simulink model "torqueBalancingR2015a"  (Simulink 8.5)
settings: Solver=FixedStepDiscrete  StartTime=0.0  StopTime="CONFIG.SIMULATION_TIME "  FixedStep=CONFIG.Ts  RelTol=1e-3
InitFcn:
  | cd(fileparts(which(bdroot)));
  | initTorqueBalancing;
values from neighbouring files (symbols this model uses):
  WBT_robotName = 'iCub'    [initTorqueBalancing.m]
undefined symbols (not defined in the file or in its folder): bVectorConstraints, CONFIG, ConstraintsMatrix, DiscIntNeverNeededParam, gain, references, reg, ROBOT_DOF, ROBOT_DOF_FOR_SIMULINK, sat, SM, sm
libraries: WBToolboxLibrary x126, simulink x6
(part 2 of 3)

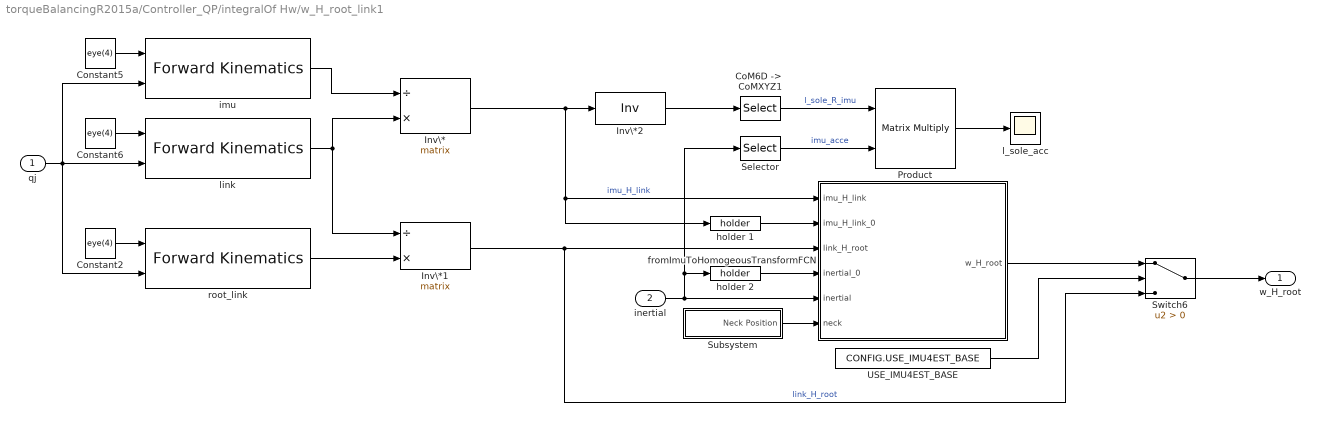
== system torqueBalancingR2015a/Controller_QP/integralOf Hw/w_H_root_link1 ==
  qj : Inport
  inertial : Inport  Port=2
  "CoM6D ->  CoMXYZ1" : Selector  NumberOfDimensions=2  InputPortWidth=7  IndexOptions=Index vector (dialog),Index vector (dialog)  Indices=[1 2 3],[1 2 3]  OutputSizes=1,1
  Constant2 : Constant  Value=eye(4)
  Constant5 : Constant  Value=eye(4)
  Constant6 : Constant  Value=eye(4)
  Inv\* : Product  Inputs=/*  Multiplication=Matrix(*)
  Inv\*1 : Product  Inputs=/*  Multiplication=Matrix(*)
  Inv\*2 : Product  Inputs=/  Multiplication=Matrix(*)
  Product : Product  Multiplication=Matrix(*)
  Selector : Selector  InputPortWidth=12  IndexOptions=Index vector (dialog)  Indices=[4 5 6 ]  OutputSizes=1
  Subsystem : Subsystem
  Switch6 : Switch  Criteria=u2 > Threshold
  USE_IMU4EST_BASE : Constant  Value=CONFIG.USE_IMU4EST_BASE
  fromImuToHomogeousTransformFCN : MATLAB Function  TreatAsAtomicUnit=on
      settings: PermitHierarchicalResolution=ParametersOnly
  holder 1 : WBToolboxLibrary/Utilities/holder 
  holder 2 : WBToolboxLibrary/Utilities/holder 
  imu : WBToolboxLibrary/wholeBodyModel/Kinematics/Forward Kinematics  frameName='imu_frame'  robotName=WBT_robotName  localName=WBT_modelName  wbiFile=WBT_wbiFilename  wbiList=WBT_wbiList
  l_sole_acc : Scope
      settings: TimeRange=auto  LimitDataPoints=on  MaxDataPoints=5000  SaveToWorkspace=off  SaveName=ScopeData  YMin=-10  YMax=10  SampleTime=-1  DataFormat=Array
  link : WBToolboxLibrary/wholeBodyModel/Kinematics/Forward Kinematics  frameName=link_name  robotName=WBT_robotName  localName=WBT_modelName  wbiFile=WBT_wbiFilename  wbiList=WBT_wbiList
  root_link : WBToolboxLibrary/wholeBodyModel/Kinematics/Forward Kinematics  frameName='root_link'  robotName=WBT_robotName  localName=WBT_modelName  wbiFile=WBT_wbiFilename  wbiList=WBT_wbiList
  w_H_root : Outport
  wires:
  Constant5/1 -> imu/1
  Inv\*/1 -> holder 1/1, fromImuToHomogeousTransformFCN/1(imu_H_link), Inv\*2/1  "imu_H_link"
  imu/1 -> Inv\*/1
  Constant6/1 -> link/1
  Inv\*1/1 -> Switch6/3, fromImuToHomogeousTransformFCN/3(link_H_root)  "link_H_root"
  link/1 -> Inv\*1/1, Inv\*/2
  inertial/1 -> Selector/1, holder 2/1, fromImuToHomogeousTransformFCN/5(inertial)
  Switch6/1 -> w_H_root/1
  USE_IMU4EST_BASE/1 -> Switch6/2
  fromImuToHomogeousTransformFCN/1(w_H_root) -> Switch6/1
  Constant2/1 -> root_link/1
  qj/1 -> root_link/2, link/2, imu/2
  root_link/1 -> Inv\*1/2
  holder 1/1 -> fromImuToHomogeousTransformFCN/2(imu_H_link_0)
  holder 2/1 -> fromImuToHomogeousTransformFCN/4(inertial_0)
  Inv\*2/1 -> "CoM6D ->  CoMXYZ1"/1
  "CoM6D ->  CoMXYZ1"/1 -> Product/1  "l_sole_R_imu"
  Selector/1 -> Product/2  "imu_acce"
  Product/1 -> l_sole_acc/1
  Subsystem/1(Neck Position) -> fromImuToHomogeousTransformFCN/6(neck)

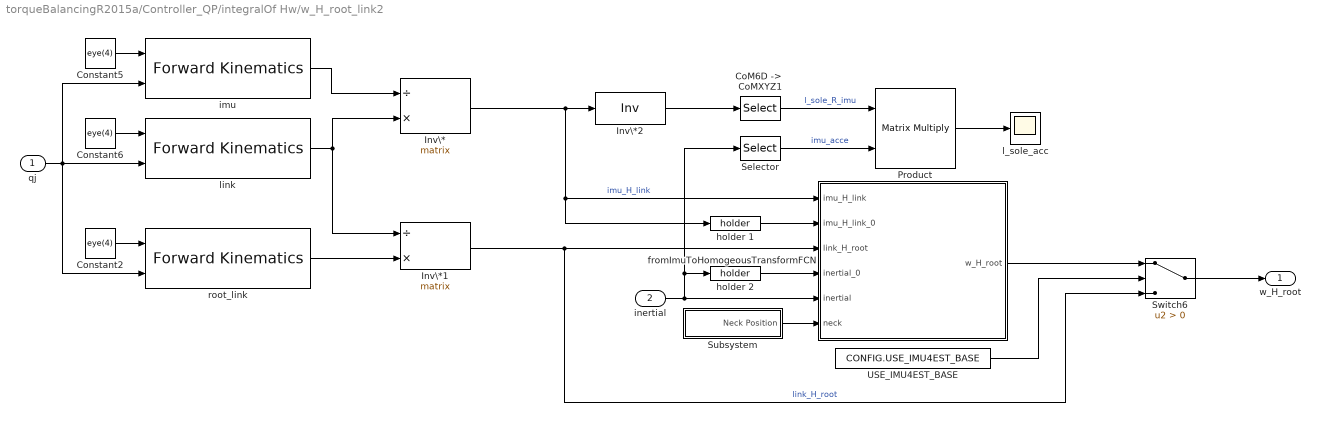
== system torqueBalancingR2015a/Controller_QP/integralOf Hw/w_H_root_link2 ==
  qj : Inport
  inertial : Inport  Port=2
  "CoM6D ->  CoMXYZ1" : Selector  NumberOfDimensions=2  InputPortWidth=7  IndexOptions=Index vector (dialog),Index vector (dialog)  Indices=[1 2 3],[1 2 3]  OutputSizes=1,1
  Constant2 : Constant  Value=eye(4)
  Constant5 : Constant  Value=eye(4)
  Constant6 : Constant  Value=eye(4)
  Inv\* : Product  Inputs=/*  Multiplication=Matrix(*)
  Inv\*1 : Product  Inputs=/*  Multiplication=Matrix(*)
  Inv\*2 : Product  Inputs=/  Multiplication=Matrix(*)
  Product : Product  Multiplication=Matrix(*)
  Selector : Selector  InputPortWidth=12  IndexOptions=Index vector (dialog)  Indices=[4 5 6 ]  OutputSizes=1
  Subsystem : Subsystem
  Switch6 : Switch  Criteria=u2 > Threshold
  USE_IMU4EST_BASE : Constant  Value=CONFIG.USE_IMU4EST_BASE
  fromImuToHomogeousTransformFCN : MATLAB Function  TreatAsAtomicUnit=on
      settings: PermitHierarchicalResolution=ParametersOnly
  holder 1 : WBToolboxLibrary/Utilities/holder 
  holder 2 : WBToolboxLibrary/Utilities/holder 
  imu : WBToolboxLibrary/wholeBodyModel/Kinematics/Forward Kinematics  frameName='imu_frame'  robotName=WBT_robotName  localName=WBT_modelName  wbiFile=WBT_wbiFilename  wbiList=WBT_wbiList
  l_sole_acc : Scope
      settings: TimeRange=auto  LimitDataPoints=on  MaxDataPoints=5000  SaveToWorkspace=off  SaveName=ScopeData  YMin=-10  YMax=10  SampleTime=-1  DataFormat=Array
  link : WBToolboxLibrary/wholeBodyModel/Kinematics/Forward Kinematics  frameName=link_name  robotName=WBT_robotName  localName=WBT_modelName  wbiFile=WBT_wbiFilename  wbiList=WBT_wbiList
  root_link : WBToolboxLibrary/wholeBodyModel/Kinematics/Forward Kinematics  frameName='root_link'  robotName=WBT_robotName  localName=WBT_modelName  wbiFile=WBT_wbiFilename  wbiList=WBT_wbiList
  w_H_root : Outport
  wires:
  Constant5/1 -> imu/1
  Inv\*/1 -> holder 1/1, fromImuToHomogeousTransformFCN/1(imu_H_link), Inv\*2/1  "imu_H_link"
  imu/1 -> Inv\*/1
  Constant6/1 -> link/1
  Inv\*1/1 -> Switch6/3, fromImuToHomogeousTransformFCN/3(link_H_root)  "link_H_root"
  link/1 -> Inv\*1/1, Inv\*/2
  inertial/1 -> Selector/1, holder 2/1, fromImuToHomogeousTransformFCN/5(inertial)
  Switch6/1 -> w_H_root/1
  USE_IMU4EST_BASE/1 -> Switch6/2
  fromImuToHomogeousTransformFCN/1(w_H_root) -> Switch6/1
  Constant2/1 -> root_link/1
  qj/1 -> root_link/2, link/2, imu/2
  root_link/1 -> Inv\*1/2
  holder 1/1 -> fromImuToHomogeousTransformFCN/2(imu_H_link_0)
  holder 2/1 -> fromImuToHomogeousTransformFCN/4(inertial_0)
  Inv\*2/1 -> "CoM6D ->  CoMXYZ1"/1
  "CoM6D ->  CoMXYZ1"/1 -> Product/1  "l_sole_R_imu"
  Selector/1 -> Product/2  "imu_acce"
  Product/1 -> l_sole_acc/1
  Subsystem/1(Neck Position) -> fromImuToHomogeousTransformFCN/6(neck)

== system torqueBalancingR2015a/State Machine/Internal coordinator/nu ==
  qj : Inport
  w_H_b : Inport  Port=2
  "constraints " : Inport  Port=3
  Get Estimate : WBToolboxLibrary/wholeBodyStates/Get Estimate  estimateType=Joints Velocity  robotName=WBT_robotName  localName=WBT_modelName  wbiFile=WBT_wbiFilename  wbiList=WBT_wbiList
  Jacobian l_sole : WBToolboxLibrary/wholeBodyModel/Jacobians/Jacobian  frameName='l_sole'  robotName=WBT_robotName  localName=WBT_modelName  wbiFile=WBT_wbiFilename  wbiList=WBT_wbiList
  Jacobian r_sole : WBToolboxLibrary/wholeBodyModel/Jacobians/Jacobian  frameName='r_sole'  robotName=WBT_robotName  localName=WBT_modelName  wbiFile=WBT_wbiFilename  wbiList=WBT_wbiList
  MATLAB Function : MATLAB Function  TreatAsAtomicUnit=on
      settings: PermitHierarchicalResolution=ParametersOnly
  Mux : Mux  Inputs=2
  vb + Dqj : Outport
  wires:
  Get Estimate/1 -> MATLAB Function/4(qD), Mux/2
  Mux/1 -> vb + Dqj/1
  Jacobian r_sole/1 -> MATLAB Function/2(JcRightFoot)
  "constraints "/1 -> MATLAB Function/3(activeFeetConstraints)
  MATLAB Function/1(y) -> Mux/1
  Jacobian l_sole/1 -> MATLAB Function/1(JcLeftFoot)
  qj/1 -> Jacobian l_sole/2, Jacobian r_sole/2
  w_H_b/1 -> Jacobian r_sole/1, Jacobian l_sole/1

== system torqueBalancingR2015a/State Machine/Internal coordinator/refGen ==
  xCom(0) : Inport
  qj(0) : Inport  Port=2
  Enable : EnablePort
  Clock1 : Clock
  refGenFCN : MATLAB Function  TreatAsAtomicUnit=on
      settings: PermitHierarchicalResolution=ParametersOnly
  qDes : Outport
  CoMrefs : Outport  Port=2
  wires:
  refGenFCN/2(desired_x_dx_ddx_CoM) -> CoMrefs/1
  xCom(0)/1 -> refGenFCN/1(xCom0)
  Clock1/1 -> refGenFCN/3(t)
  qj(0)/1 -> refGenFCN/2(q0)
  refGenFCN/1(qDes) -> qDes/1

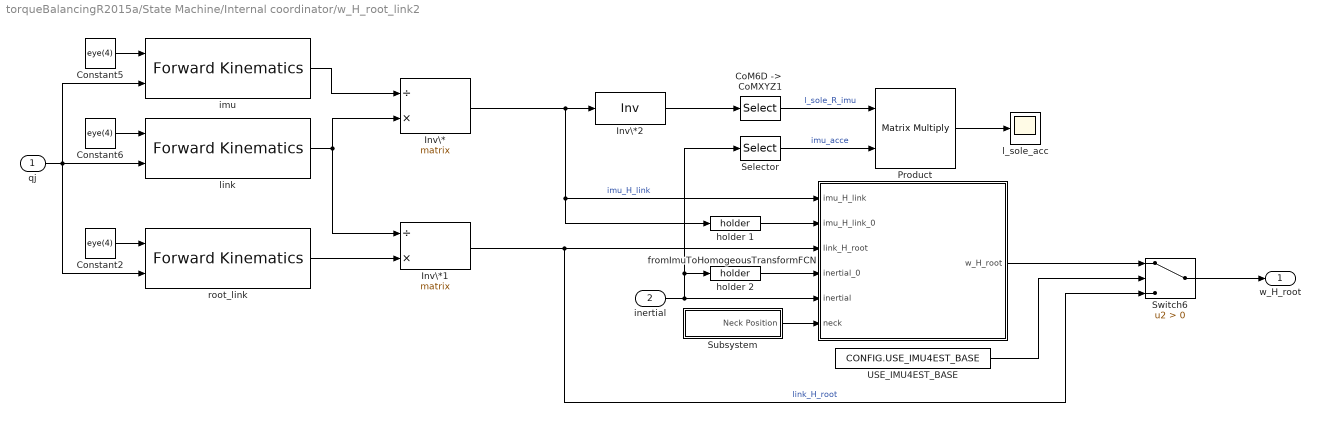
== system torqueBalancingR2015a/State Machine/Internal coordinator/w_H_root_link2 ==
  qj : Inport
  inertial : Inport  Port=2
  "CoM6D ->  CoMXYZ1" : Selector  NumberOfDimensions=2  InputPortWidth=7  IndexOptions=Index vector (dialog),Index vector (dialog)  Indices=[1 2 3],[1 2 3]  OutputSizes=1,1
  Constant2 : Constant  Value=eye(4)
  Constant5 : Constant  Value=eye(4)
  Constant6 : Constant  Value=eye(4)
  Inv\* : Product  Inputs=/*  Multiplication=Matrix(*)
  Inv\*1 : Product  Inputs=/*  Multiplication=Matrix(*)
  Inv\*2 : Product  Inputs=/  Multiplication=Matrix(*)
  Product : Product  Multiplication=Matrix(*)
  Selector : Selector  InputPortWidth=12  IndexOptions=Index vector (dialog)  Indices=[4 5 6 ]  OutputSizes=1
  Subsystem : Subsystem
  Switch6 : Switch  Criteria=u2 > Threshold
  USE_IMU4EST_BASE : Constant  Value=CONFIG.USE_IMU4EST_BASE
  fromImuToHomogeousTransformFCN : MATLAB Function  TreatAsAtomicUnit=on
      settings: PermitHierarchicalResolution=ParametersOnly
  holder 1 : WBToolboxLibrary/Utilities/holder 
  holder 2 : WBToolboxLibrary/Utilities/holder 
  imu : WBToolboxLibrary/wholeBodyModel/Kinematics/Forward Kinematics  frameName='imu_frame'  robotName=WBT_robotName  localName=WBT_modelName  wbiFile=WBT_wbiFilename  wbiList=WBT_wbiList
  l_sole_acc : Scope
      settings: TimeRange=auto  LimitDataPoints=on  MaxDataPoints=5000  SaveToWorkspace=off  SaveName=ScopeData  YMin=-10  YMax=10  SampleTime=-1  DataFormat=Array
  link : WBToolboxLibrary/wholeBodyModel/Kinematics/Forward Kinematics  frameName=link_name  robotName=WBT_robotName  localName=WBT_modelName  wbiFile=WBT_wbiFilename  wbiList=WBT_wbiList
  root_link : WBToolboxLibrary/wholeBodyModel/Kinematics/Forward Kinematics  frameName='root_link'  robotName=WBT_robotName  localName=WBT_modelName  wbiFile=WBT_wbiFilename  wbiList=WBT_wbiList
  w_H_root : Outport
  wires:
  Constant5/1 -> imu/1
  Inv\*/1 -> holder 1/1, fromImuToHomogeousTransformFCN/1(imu_H_link), Inv\*2/1  "imu_H_link"
  imu/1 -> Inv\*/1
  Constant6/1 -> link/1
  Inv\*1/1 -> Switch6/3, fromImuToHomogeousTransformFCN/3(link_H_root)  "link_H_root"
  link/1 -> Inv\*1/1, Inv\*/2
  inertial/1 -> Selector/1, holder 2/1, fromImuToHomogeousTransformFCN/5(inertial)
  Switch6/1 -> w_H_root/1
  USE_IMU4EST_BASE/1 -> Switch6/2
  fromImuToHomogeousTransformFCN/1(w_H_root) -> Switch6/1
  Constant2/1 -> root_link/1
  qj/1 -> root_link/2, link/2, imu/2
  root_link/1 -> Inv\*1/2
  holder 1/1 -> fromImuToHomogeousTransformFCN/2(imu_H_link_0)
  holder 2/1 -> fromImuToHomogeousTransformFCN/4(inertial_0)
  Inv\*2/1 -> "CoM6D ->  CoMXYZ1"/1
  "CoM6D ->  CoMXYZ1"/1 -> Product/1  "l_sole_R_imu"
  Selector/1 -> Product/2  "imu_acce"
  Product/1 -> l_sole_acc/1
  Subsystem/1(Neck Position) -> fromImuToHomogeousTransformFCN/6(neck)

== system torqueBalancingR2015a/State Machine/Internal coordinator/xCom ==
  w_H_b : Inport
  qj : Inport  Port=2
  "CoM6D ->  CoMXYZ2" : Selector  NumberOfDimensions=2  InputPortWidth=7  IndexOptions=Index vector (dialog),Index vector (dialog)  Indices=[1 2 3],[4]  OutputSizes=1,1
  com : WBToolboxLibrary/wholeBodyModel/Kinematics/Forward Kinematics  frameName='com'  robotName=WBT_robotName  localName=WBT_modelName  wbiFile=WBT_wbiFilename  wbiList=WBT_wbiList
  xCom : Outport
  wires:
  qj/1 -> com/2
  "CoM6D ->  CoMXYZ2"/1 -> xCom/1
  com/1 -> "CoM6D ->  CoMXYZ2"/1
  w_H_b/1 -> com/1

== system torqueBalancingR2015a/State Machine/State Machine Walking/Visualise external wrenches   ==
  wL_WBDT : Inport
  wR_WBDT : Inport  Port=2
  Enable : EnablePort
  Constant : Constant  Value=sm.wrench.thresholdContactOn
  Constant2 : Constant  Value=sm.wrench.thresholdContactOff
  left foot ext wrench : Scope  NumInputPorts=3
      settings: TimeRange=auto  LimitDataPoints=on  MaxDataPoints=5000  SaveToWorkspace=off  SaveName=ScopeData  YMin=-47.59687~15.00000~75.00000  YMax=331.67201~35.00000~95.00000  SampleTime=-1  DataFormat=Array
  right foot ext wrench : Scope  NumInputPorts=3
      settings: TimeRange=auto  LimitDataPoints=on  MaxDataPoints=5000  SaveToWorkspace=off  SaveName=ScopeData  YMin=-42.03924~15.00000~75.00000  YMax=233.22188~35.00000~95.00000  SampleTime=-1  DataFormat=Array
  wires:
  Constant/1 -> right foot ext wrench/2, left foot ext wrench/2  "thresholdContactOn"
  wR_WBDT/1 -> right foot ext wrench/1  "wR_WBDT"
  wL_WBDT/1 -> left foot ext wrench/1  "wL_WBDT"
  Constant2/1 -> right foot ext wrench/3, left foot ext wrench/3  "thresholdContactOff"

== system torqueBalancingR2015a/State Machine/State Machine Walking/nu ==
  w_H_b : Inport
  "constraints " : Inport  Port=2
  qj : Inport  Port=3
  Get Estimate : WBToolboxLibrary/wholeBodyStates/Get Estimate  estimateType=Joints Velocity  robotName=WBT_robotName  localName=WBT_modelName  wbiFile=WBT_wbiFilename  wbiList=WBT_wbiList
  Jacobian l_sole : WBToolboxLibrary/wholeBodyModel/Jacobians/Jacobian  frameName='l_sole'  robotName=WBT_robotName  localName=WBT_modelName  wbiFile=WBT_wbiFilename  wbiList=WBT_wbiList
  Jacobian r_sole : WBToolboxLibrary/wholeBodyModel/Jacobians/Jacobian  frameName='r_sole'  robotName=WBT_robotName  localName=WBT_modelName  wbiFile=WBT_wbiFilename  wbiList=WBT_wbiList
  MATLAB Function : MATLAB Function  TreatAsAtomicUnit=on
      settings: PermitHierarchicalResolution=ParametersOnly
  Mux : Mux  Inputs=2
  vb + Dqj : Outport
  wires:
  Get Estimate/1 -> MATLAB Function/4(qD), Mux/2
  Mux/1 -> vb + Dqj/1
  Jacobian r_sole/1 -> MATLAB Function/2(JcRightFoot)
  "constraints "/1 -> MATLAB Function/3(activeFeetConstraints)
  MATLAB Function/1(y) -> Mux/1
  Jacobian l_sole/1 -> MATLAB Function/1(JcLeftFoot)
  qj/1 -> Jacobian l_sole/2, Jacobian r_sole/2
  w_H_b/1 -> Jacobian r_sole/1, Jacobian l_sole/1

== system torqueBalancingR2015a/State Machine/State Machine Walking/visualise inertial ==
  jointAngles : Inport
  inertial : Inport  Port=2
  Enable : EnablePort
  Inv\* : Product  Inputs=/*  Multiplication=Matrix(*)
  Inv\*1 : Product  Inputs=/*  Multiplication=Matrix(*)
  Visualize hom transf1 : Subsystem
  Visualize hom transf2 : Subsystem
  Visualize hom transf3 : Subsystem
  Visualize hom transf4 : Subsystem
  Visualize hom transf5 : Subsystem
  Visualize hom transf7 : Subsystem
  "inertial -> rpy" : Selector  InputPortWidth=12  IndexOptions=Index vector (dialog)  Indices=[1 2 3]  OutputSizes=1
  l_sole_H_root_link1 : Subsystem  mask{link_name='l_sole'}
  l_sole_H_root_link2 : Subsystem  mask{link_name='l_sole'}
  rpy : Scope
      settings: TimeRange=auto  LimitDataPoints=on  MaxDataPoints=5000  SaveToWorkspace=off  SaveName=ScopeData  YMin=-10  YMax=10  SampleTime=-1  DataFormat=Array
  w_H_root_link1 : Subsystem  mask{link_name='r_sole'}
      mask prompts: link_name "link name"
      mask help:
      | This block evaluates the homogeneous transformation between the world and the root link, i.e. ^wH_b. It assumes that the link specified by the variable 'link_name' has a constant position
      | w.r.t. an inertial frame, but it can rotate arbitrarily. This rotation is retrived from the IMU sensor.
      mask Display:
      | str = strrep(link_name, '_','\_');
      | port_label('output',1,['{}^{',str '}H_{root}'],'texmode','on')
      | clear str;
      | 
      | port_label('input',1,'q_j','texmode','on')
      | 
      | port_label('input',2,'inertial','texmode','on')
  w_H_root_link2 : Subsystem  mask{link_name='l_sole'}
      mask prompts: link_name "link name"
      mask help:
      | This block evaluates the homogeneous transformation between the world and the root link, i.e. ^wH_b. It assumes that the link specified by the variable 'link_name' has a constant position
      | w.r.t. an inertial frame, but it can rotate arbitrarily. This rotation is retrived from the IMU sensor.
      mask Display:
      | str = strrep(link_name, '_','\_');
      | port_label('output',1,['{}^{',str '}H_{root}'],'texmode','on')
      | clear str;
      | 
      | port_label('input',1,'q_j','texmode','on')
      | 
      | port_label('input',2,'inertial','texmode','on')
  wires:
  inertial/1 -> w_H_root_link1/2(inertial), w_H_root_link2/2(inertial), "inertial -> rpy"/1
  jointAngles/1 -> l_sole_H_root_link2/1(qj), l_sole_H_root_link1/1(qj), w_H_root_link1/1(qj), w_H_root_link2/1(qj)
  l_sole_H_root_link2/1(link_name_H_root_link) -> Visualize hom transf7/1(H), Inv\*/1  "l_sole_H_root_link"
  Inv\*/1 -> Visualize hom transf4/1(H)
  w_H_root_link2/1(w_H_root) -> Inv\*/2, Visualize hom transf1/1(H)
  "inertial -> rpy"/1 -> rpy/1
  l_sole_H_root_link1/1(link_name_H_root_link) -> Visualize hom transf2/1(H), Inv\*1/1  "r_sole_H_root_link"
  Inv\*1/1 -> Visualize hom transf3/1(H)
  w_H_root_link1/1(w_H_root) -> Inv\*1/2, Visualize hom transf5/1(H)

== system torqueBalancingR2015a/State Machine/State Machine Walking/xCom2 ==
  qj : Inport
  w_H_b : Inport  Port=2
  "CoM6D ->  CoMXYZ2" : Selector  NumberOfDimensions=2  InputPortWidth=7  IndexOptions=Index vector (dialog),Index vector (dialog)  Indices=[1 2 3],[4]  OutputSizes=1,1
  com : WBToolboxLibrary/wholeBodyModel/Kinematics/Forward Kinematics  frameName='com'  robotName=WBT_robotName  localName=WBT_modelName  wbiFile=WBT_wbiFilename  wbiList=WBT_wbiList
  xCoM : Outport
  wires:
  qj/1 -> com/2
  "CoM6D ->  CoMXYZ2"/1 -> xCoM/1
  com/1 -> "CoM6D ->  CoMXYZ2"/1
  w_H_b/1 -> com/1

== system torqueBalancingR2015a/State Machine/State Machine Yoga/Visualise external wrenches   ==
  wL_WBDT : Inport
  wR_WBDT : Inport  Port=2
  Enable : EnablePort
  Constant : Constant  Value=sm.wrench.thresholdContactOn
  Constant2 : Constant  Value=sm.wrench.thresholdContactOff
  left foot ext wrench : Scope  NumInputPorts=3
      settings: TimeRange=auto  LimitDataPoints=on  MaxDataPoints=5000  SaveToWorkspace=off  SaveName=ScopeData  YMin=-10~-10~-10  YMax=10~10~10  SampleTime=-1  DataFormat=Array
  right foot ext wrench : Scope  NumInputPorts=3
      settings: TimeRange=auto  LimitDataPoints=on  MaxDataPoints=5000  SaveToWorkspace=off  SaveName=ScopeData  YMin=-10~-10~-10  YMax=10~10~10  SampleTime=-1  DataFormat=Array
  wires:
  Constant/1 -> left foot ext wrench/2, right foot ext wrench/2  "thresholdContactOn"
  wR_WBDT/1 -> right foot ext wrench/1  "wR_WBDT"
  wL_WBDT/1 -> left foot ext wrench/1  "wL_WBDT"
  Constant2/1 -> left foot ext wrench/3, right foot ext wrench/3  "thresholdContactOff"

== system torqueBalancingR2015a/State Machine/State Machine Yoga/nu ==
  qj : Inport
  w_H_b : Inport  Port=2
  "constraints " : Inport  Port=3
  Get Estimate : WBToolboxLibrary/wholeBodyStates/Get Estimate  estimateType=Joints Velocity  robotName=WBT_robotName  localName=WBT_modelName  wbiFile=WBT_wbiFilename  wbiList=WBT_wbiList
  Jacobian l_sole : WBToolboxLibrary/wholeBodyModel/Jacobians/Jacobian  frameName='l_sole'  robotName=WBT_robotName  localName=WBT_modelName  wbiFile=WBT_wbiFilename  wbiList=WBT_wbiList
  Jacobian r_sole : WBToolboxLibrary/wholeBodyModel/Jacobians/Jacobian  frameName='r_sole'  robotName=WBT_robotName  localName=WBT_modelName  wbiFile=WBT_wbiFilename  wbiList=WBT_wbiList
  MATLAB Function : MATLAB Function  TreatAsAtomicUnit=on
      settings: PermitHierarchicalResolution=ParametersOnly
  Mux : Mux  Inputs=2
  vb + Dqj : Outport
  wires:
  Get Estimate/1 -> MATLAB Function/4(qD), Mux/2
  Mux/1 -> vb + Dqj/1
  Jacobian r_sole/1 -> MATLAB Function/2(JcRightFoot)
  "constraints "/1 -> MATLAB Function/3(activeFeetConstraints)
  MATLAB Function/1(y) -> Mux/1
  Jacobian l_sole/1 -> MATLAB Function/1(JcLeftFoot)
  qj/1 -> Jacobian l_sole/2, Jacobian r_sole/2
  w_H_b/1 -> Jacobian r_sole/1, Jacobian l_sole/1

== system torqueBalancingR2015a/State Machine/State Machine Yoga/visualise inertial ==
  jointAngles : Inport
  inertial : Inport  Port=2
  Enable : EnablePort
  Inv\* : Product  Inputs=/*  Multiplication=Matrix(*)
  Inv\*1 : Product  Inputs=/*  Multiplication=Matrix(*)
  Visualize hom transf1 : Subsystem
  Visualize hom transf2 : Subsystem
  Visualize hom transf3 : Subsystem
  Visualize hom transf4 : Subsystem
  Visualize hom transf5 : Subsystem
  Visualize hom transf7 : Subsystem
  "inertial -> rpy" : Selector  InputPortWidth=12  IndexOptions=Index vector (dialog)  Indices=[1 2 3]  OutputSizes=1
  l_sole_H_root_link1 : Subsystem  mask{link_name='l_sole'}
  l_sole_H_root_link2 : Subsystem  mask{link_name='l_sole'}
  rpy : Scope
      settings: TimeRange=auto  LimitDataPoints=on  MaxDataPoints=5000  SaveToWorkspace=off  SaveName=ScopeData  YMin=-10  YMax=10  SampleTime=-1  DataFormat=Array
  w_H_root_link1 : Subsystem  mask{link_name='r_sole'}
      mask prompts: link_name "link name"
      mask help:
      | This block evaluates the homogeneous transformation between the world and the root link, i.e. ^wH_b. It assumes that the link specified by the variable 'link_name' has a constant position
      | w.r.t. an inertial frame, but it can rotate arbitrarily. This rotation is retrived from the IMU sensor.
      mask Display:
      | str = strrep(link_name, '_','\_');
      | port_label('output',1,['{}^{',str '}H_{root}'],'texmode','on')
      | clear str;
      | 
      | port_label('input',1,'q_j','texmode','on')
      | 
      | port_label('input',2,'inertial','texmode','on')
  w_H_root_link2 : Subsystem  mask{link_name='l_sole'}
      mask prompts: link_name "link name"
      mask help:
      | This block evaluates the homogeneous transformation between the world and the root link, i.e. ^wH_b. It assumes that the link specified by the variable 'link_name' has a constant position
      | w.r.t. an inertial frame, but it can rotate arbitrarily. This rotation is retrived from the IMU sensor.
      mask Display:
      | str = strrep(link_name, '_','\_');
      | port_label('output',1,['{}^{',str '}H_{root}'],'texmode','on')
      | clear str;
      | 
      | port_label('input',1,'q_j','texmode','on')
      | 
      | port_label('input',2,'inertial','texmode','on')
  wires:
  inertial/1 -> w_H_root_link1/2(inertial), w_H_root_link2/2(inertial), "inertial -> rpy"/1
  jointAngles/1 -> l_sole_H_root_link2/1(qj), l_sole_H_root_link1/1(qj), w_H_root_link1/1(qj), w_H_root_link2/1(qj)
  l_sole_H_root_link2/1(link_name_H_root_link) -> Visualize hom transf7/1(H), Inv\*/1  "l_sole_H_root_link"
  Inv\*/1 -> Visualize hom transf4/1(H)
  w_H_root_link2/1(w_H_root) -> Inv\*/2, Visualize hom transf1/1(H)
  "inertial -> rpy"/1 -> rpy/1
  l_sole_H_root_link1/1(link_name_H_root_link) -> Visualize hom transf2/1(H), Inv\*1/1  "r_sole_H_root_link"
  Inv\*1/1 -> Visualize hom transf3/1(H)
  w_H_root_link1/1(w_H_root) -> Inv\*1/2, Visualize hom transf5/1(H)

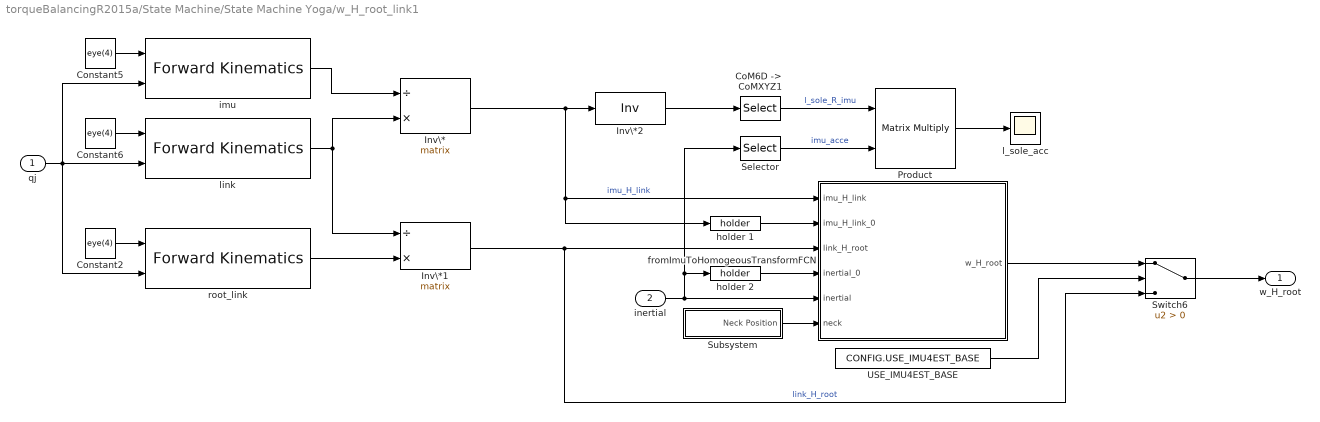
== system torqueBalancingR2015a/State Machine/State Machine Yoga/w_H_root_link1 ==
  qj : Inport
  inertial : Inport  Port=2
  "CoM6D ->  CoMXYZ1" : Selector  NumberOfDimensions=2  InputPortWidth=7  IndexOptions=Index vector (dialog),Index vector (dialog)  Indices=[1 2 3],[1 2 3]  OutputSizes=1,1
  Constant2 : Constant  Value=eye(4)
  Constant5 : Constant  Value=eye(4)
  Constant6 : Constant  Value=eye(4)
  Inv\* : Product  Inputs=/*  Multiplication=Matrix(*)
  Inv\*1 : Product  Inputs=/*  Multiplication=Matrix(*)
  Inv\*2 : Product  Inputs=/  Multiplication=Matrix(*)
  Product : Product  Multiplication=Matrix(*)
  Selector : Selector  InputPortWidth=12  IndexOptions=Index vector (dialog)  Indices=[4 5 6 ]  OutputSizes=1
  Subsystem : Subsystem
  Switch6 : Switch  Criteria=u2 > Threshold
  USE_IMU4EST_BASE : Constant  Value=CONFIG.USE_IMU4EST_BASE
  fromImuToHomogeousTransformFCN : MATLAB Function  TreatAsAtomicUnit=on
      settings: PermitHierarchicalResolution=ParametersOnly
  holder 1 : WBToolboxLibrary/Utilities/holder 
  holder 2 : WBToolboxLibrary/Utilities/holder 
  imu : WBToolboxLibrary/wholeBodyModel/Kinematics/Forward Kinematics  frameName='imu_frame'  robotName=WBT_robotName  localName=WBT_modelName  wbiFile=WBT_wbiFilename  wbiList=WBT_wbiList
  l_sole_acc : Scope
      settings: TimeRange=auto  LimitDataPoints=on  MaxDataPoints=5000  SaveToWorkspace=off  SaveName=ScopeData  YMin=-10  YMax=10  SampleTime=-1  DataFormat=Array
  link : WBToolboxLibrary/wholeBodyModel/Kinematics/Forward Kinematics  frameName=link_name  robotName=WBT_robotName  localName=WBT_modelName  wbiFile=WBT_wbiFilename  wbiList=WBT_wbiList
  root_link : WBToolboxLibrary/wholeBodyModel/Kinematics/Forward Kinematics  frameName='root_link'  robotName=WBT_robotName  localName=WBT_modelName  wbiFile=WBT_wbiFilename  wbiList=WBT_wbiList
  w_H_root : Outport
  wires:
  Constant5/1 -> imu/1
  Inv\*/1 -> holder 1/1, fromImuToHomogeousTransformFCN/1(imu_H_link), Inv\*2/1  "imu_H_link"
  imu/1 -> Inv\*/1
  Constant6/1 -> link/1
  Inv\*1/1 -> Switch6/3, fromImuToHomogeousTransformFCN/3(link_H_root)  "link_H_root"
  link/1 -> Inv\*1/1, Inv\*/2
  inertial/1 -> Selector/1, holder 2/1, fromImuToHomogeousTransformFCN/5(inertial)
  Switch6/1 -> w_H_root/1
  USE_IMU4EST_BASE/1 -> Switch6/2
  fromImuToHomogeousTransformFCN/1(w_H_root) -> Switch6/1
  Constant2/1 -> root_link/1
  qj/1 -> root_link/2, link/2, imu/2
  root_link/1 -> Inv\*1/2
  holder 1/1 -> fromImuToHomogeousTransformFCN/2(imu_H_link_0)
  holder 2/1 -> fromImuToHomogeousTransformFCN/4(inertial_0)
  Inv\*2/1 -> "CoM6D ->  CoMXYZ1"/1
  "CoM6D ->  CoMXYZ1"/1 -> Product/1  "l_sole_R_imu"
  Selector/1 -> Product/2  "imu_acce"
  Product/1 -> l_sole_acc/1
  Subsystem/1(Neck Position) -> fromImuToHomogeousTransformFCN/6(neck)

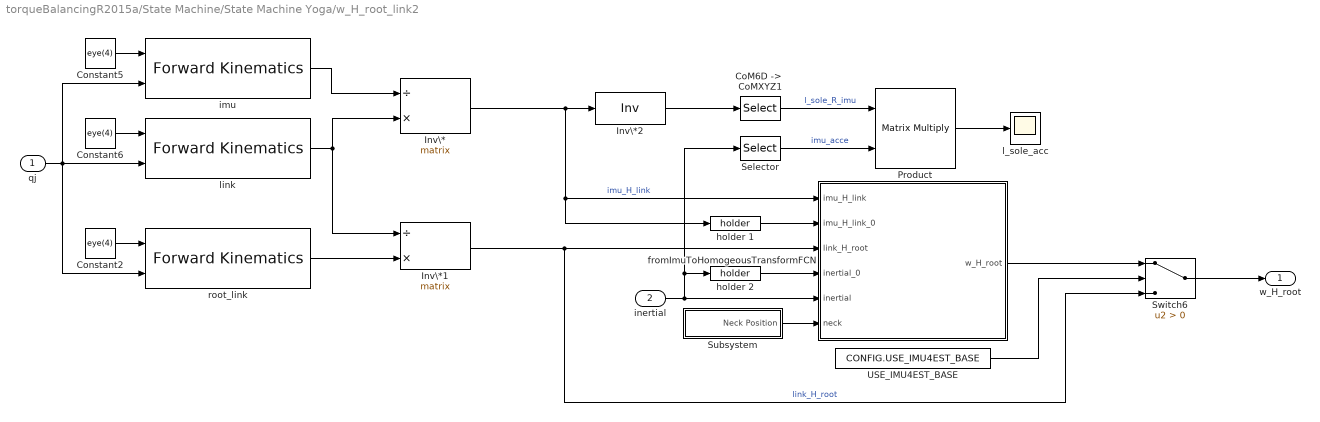
== system torqueBalancingR2015a/State Machine/State Machine Yoga/w_H_root_link2 ==
  qj : Inport
  inertial : Inport  Port=2
  "CoM6D ->  CoMXYZ1" : Selector  NumberOfDimensions=2  InputPortWidth=7  IndexOptions=Index vector (dialog),Index vector (dialog)  Indices=[1 2 3],[1 2 3]  OutputSizes=1,1
  Constant2 : Constant  Value=eye(4)
  Constant5 : Constant  Value=eye(4)
  Constant6 : Constant  Value=eye(4)
  Inv\* : Product  Inputs=/*  Multiplication=Matrix(*)
  Inv\*1 : Product  Inputs=/*  Multiplication=Matrix(*)
  Inv\*2 : Product  Inputs=/  Multiplication=Matrix(*)
  Product : Product  Multiplication=Matrix(*)
  Selector : Selector  InputPortWidth=12  IndexOptions=Index vector (dialog)  Indices=[4 5 6 ]  OutputSizes=1
  Subsystem : Subsystem
  Switch6 : Switch  Criteria=u2 > Threshold
  USE_IMU4EST_BASE : Constant  Value=CONFIG.USE_IMU4EST_BASE
  fromImuToHomogeousTransformFCN : MATLAB Function  TreatAsAtomicUnit=on
      settings: PermitHierarchicalResolution=ParametersOnly
  holder 1 : WBToolboxLibrary/Utilities/holder 
  holder 2 : WBToolboxLibrary/Utilities/holder 
  imu : WBToolboxLibrary/wholeBodyModel/Kinematics/Forward Kinematics  frameName='imu_frame'  robotName=WBT_robotName  localName=WBT_modelName  wbiFile=WBT_wbiFilename  wbiList=WBT_wbiList
  l_sole_acc : Scope
      settings: TimeRange=auto  LimitDataPoints=on  MaxDataPoints=5000  SaveToWorkspace=off  SaveName=ScopeData  YMin=-10  YMax=10  SampleTime=-1  DataFormat=Array
  link : WBToolboxLibrary/wholeBodyModel/Kinematics/Forward Kinematics  frameName=link_name  robotName=WBT_robotName  localName=WBT_modelName  wbiFile=WBT_wbiFilename  wbiList=WBT_wbiList
  root_link : WBToolboxLibrary/wholeBodyModel/Kinematics/Forward Kinematics  frameName='root_link'  robotName=WBT_robotName  localName=WBT_modelName  wbiFile=WBT_wbiFilename  wbiList=WBT_wbiList
  w_H_root : Outport
  wires:
  Constant5/1 -> imu/1
  Inv\*/1 -> holder 1/1, fromImuToHomogeousTransformFCN/1(imu_H_link), Inv\*2/1  "imu_H_link"
  imu/1 -> Inv\*/1
  Constant6/1 -> link/1
  Inv\*1/1 -> Switch6/3, fromImuToHomogeousTransformFCN/3(link_H_root)  "link_H_root"
  link/1 -> Inv\*1/1, Inv\*/2
  inertial/1 -> Selector/1, holder 2/1, fromImuToHomogeousTransformFCN/5(inertial)
  Switch6/1 -> w_H_root/1
  USE_IMU4EST_BASE/1 -> Switch6/2
  fromImuToHomogeousTransformFCN/1(w_H_root) -> Switch6/1
  Constant2/1 -> root_link/1
  qj/1 -> root_link/2, link/2, imu/2
  root_link/1 -> Inv\*1/2
  holder 1/1 -> fromImuToHomogeousTransformFCN/2(imu_H_link_0)
  holder 2/1 -> fromImuToHomogeousTransformFCN/4(inertial_0)
  Inv\*2/1 -> "CoM6D ->  CoMXYZ1"/1
  "CoM6D ->  CoMXYZ1"/1 -> Product/1  "l_sole_R_imu"
  Selector/1 -> Product/2  "imu_acce"
  Product/1 -> l_sole_acc/1
  Subsystem/1(Neck Position) -> fromImuToHomogeousTransformFCN/6(neck)

== system torqueBalancingR2015a/State Machine/State Machine Yoga/xCom ==
  qj : Inport
  w_H_b : Inport  Port=2
  "CoM6D ->  CoMXYZ2" : Selector  NumberOfDimensions=2  InputPortWidth=7  IndexOptions=Index vector (dialog),Index vector (dialog)  Indices=[1 2 3],[4]  OutputSizes=1,1
  com : WBToolboxLibrary/wholeBodyModel/Kinematics/Forward Kinematics  frameName='com'  robotName=WBT_robotName  localName=WBT_modelName  wbiFile=WBT_wbiFilename  wbiList=WBT_wbiList
  xCom : Outport
  wires:
  qj/1 -> com/2
  "CoM6D ->  CoMXYZ2"/1 -> xCom/1
  com/1 -> "CoM6D ->  CoMXYZ2"/1
  w_H_b/1 -> com/1

== system torqueBalancingR2015a/State Machine/State Machine Yoga/xCom1 ==
  qj : Inport
  w_H_b : Inport  Port=2
  "CoM6D ->  CoMXYZ2" : Selector  NumberOfDimensions=2  InputPortWidth=7  IndexOptions=Index vector (dialog),Index vector (dialog)  Indices=[1 2 3],[4]  OutputSizes=1,1
  com : WBToolboxLibrary/wholeBodyModel/Kinematics/Forward Kinematics  frameName='com'  robotName=WBT_robotName  localName=WBT_modelName  wbiFile=WBT_wbiFilename  wbiList=WBT_wbiList
  xCom : Outport
  wires:
  qj/1 -> com/2
  "CoM6D ->  CoMXYZ2"/1 -> xCom/1
  com/1 -> "CoM6D ->  CoMXYZ2"/1
  w_H_b/1 -> com/1

== system torqueBalancingR2015a/Controller_QP/integralOf Hw/w_H_root_link1/Subsystem ==
  Constant : Constant  Value=zeros(3,1)
  Gain : Gain  Gain=pi/180
  Head state : WBToolboxLibrary/Utilities/Yarp Read  portName=['/',WBT_robotName, '/head/state:o']  signalSize=6  blocking=off  timestamp=off  autoconnect=on  errorOnConnection=off
  Selector1 : Selector  InputPortWidth=6  IndexOptions=Index vector (dialog)  Indices=[1:3]  OutputSizes=1
  Switch : Switch  Criteria=u2 > Threshold
  USE_IMU4EST_BASE1 : Constant  Value=CONFIG.CORRECT_NECK_IMU
  Neck Position : Outport
  wires:
  Head state/1 -> Gain/1
  Selector1/1 -> Switch/1  "neck"
  USE_IMU4EST_BASE1/1 -> Switch/2
  Switch/1 -> Neck Position/1
  Gain/1 -> Selector1/1
  Constant/1 -> Switch/3

== system torqueBalancingR2015a/Controller_QP/integralOf Hw/w_H_root_link2/Subsystem ==
  Constant : Constant  Value=zeros(3,1)
  Gain : Gain  Gain=pi/180
  Head state : WBToolboxLibrary/Utilities/Yarp Read  portName=['/',WBT_robotName, '/head/state:o']  signalSize=6  blocking=off  timestamp=off  autoconnect=on  errorOnConnection=off
  Selector1 : Selector  InputPortWidth=6  IndexOptions=Index vector (dialog)  Indices=[1:3]  OutputSizes=1
  Switch : Switch  Criteria=u2 > Threshold
  USE_IMU4EST_BASE1 : Constant  Value=CONFIG.CORRECT_NECK_IMU
  Neck Position : Outport
  wires:
  Head state/1 -> Gain/1
  Selector1/1 -> Switch/1  "neck"
  USE_IMU4EST_BASE1/1 -> Switch/2
  Switch/1 -> Neck Position/1
  Gain/1 -> Selector1/1
  Constant/1 -> Switch/3

== system torqueBalancingR2015a/State Machine/Internal coordinator/w_H_root_link2/Subsystem ==
  Constant : Constant  Value=zeros(3,1)
  Gain : Gain  Gain=pi/180
  Head state : WBToolboxLibrary/Utilities/Yarp Read  portName=['/',WBT_robotName, '/head/state:o']  signalSize=6  blocking=off  timestamp=off  autoconnect=on  errorOnConnection=off
  Selector1 : Selector  InputPortWidth=6  IndexOptions=Index vector (dialog)  Indices=[1:3]  OutputSizes=1
  Switch : Switch  Criteria=u2 > Threshold
  USE_IMU4EST_BASE1 : Constant  Value=CONFIG.CORRECT_NECK_IMU
  Neck Position : Outport
  wires:
  Head state/1 -> Gain/1
  Selector1/1 -> Switch/1  "neck"
  USE_IMU4EST_BASE1/1 -> Switch/2
  Switch/1 -> Neck Position/1
  Gain/1 -> Selector1/1
  Constant/1 -> Switch/3

== system torqueBalancingR2015a/State Machine/State Machine Walking/visualise inertial/Visualize hom transf1 ==
  H : Inport
  "CoM6D ->  CoMXYZ1" : Selector  NumberOfDimensions=2  InputPortWidth=7  IndexOptions=Index vector (dialog),Index vector (dialog)  Indices=[1 2 3],[1 2 3]  OutputSizes=1,1
  "CoM6D ->  CoMXYZ2" : Selector  NumberOfDimensions=2  InputPortWidth=7  IndexOptions=Index vector (dialog),Index vector (dialog)  Indices=[1 2 3],[4]  OutputSizes=1,1
  Hom : Scope
      settings: TimeRange=auto  LimitDataPoints=on  MaxDataPoints=5000  SaveToWorkspace=off  SaveName=ScopeData  YMin=-10  YMax=10  SampleTime=-1  DataFormat=Array
  R : Scope
      settings: TimeRange=auto  LimitDataPoints=on  MaxDataPoints=5000  SaveToWorkspace=off  SaveName=ScopeData  YMin=-10  YMax=10  SampleTime=-1  DataFormat=Array
  p : Scope
      settings: TimeRange=auto  LimitDataPoints=on  MaxDataPoints=5000  SaveToWorkspace=off  SaveName=ScopeData  YMin=-10  YMax=10  SampleTime=-1  DataFormat=Array
  wires:
  "CoM6D ->  CoMXYZ1"/1 -> R/1
  "CoM6D ->  CoMXYZ2"/1 -> p/1
  H/1 -> "CoM6D ->  CoMXYZ2"/1, Hom/1, "CoM6D ->  CoMXYZ1"/1

== system torqueBalancingR2015a/State Machine/State Machine Walking/visualise inertial/Visualize hom transf2 ==
  H : Inport
  "CoM6D ->  CoMXYZ1" : Selector  NumberOfDimensions=2  InputPortWidth=7  IndexOptions=Index vector (dialog),Index vector (dialog)  Indices=[1 2 3],[1 2 3]  OutputSizes=1,1
  "CoM6D ->  CoMXYZ2" : Selector  NumberOfDimensions=2  InputPortWidth=7  IndexOptions=Index vector (dialog),Index vector (dialog)  Indices=[1 2 3],[4]  OutputSizes=1,1
  Hom : Scope
      settings: TimeRange=auto  LimitDataPoints=on  MaxDataPoints=5000  SaveToWorkspace=off  SaveName=ScopeData  YMin=-10  YMax=10  SampleTime=-1  DataFormat=Array
  R : Scope
      settings: TimeRange=auto  LimitDataPoints=on  MaxDataPoints=5000  SaveToWorkspace=off  SaveName=ScopeData  YMin=-10  YMax=10  SampleTime=-1  DataFormat=Array
  p : Scope
      settings: TimeRange=auto  LimitDataPoints=on  MaxDataPoints=5000  SaveToWorkspace=off  SaveName=ScopeData  YMin=-10  YMax=10  SampleTime=-1  DataFormat=Array
  wires:
  "CoM6D ->  CoMXYZ1"/1 -> R/1
  "CoM6D ->  CoMXYZ2"/1 -> p/1
  H/1 -> "CoM6D ->  CoMXYZ2"/1, Hom/1, "CoM6D ->  CoMXYZ1"/1

== system torqueBalancingR2015a/State Machine/State Machine Walking/visualise inertial/Visualize hom transf3 ==
  H : Inport
  "CoM6D ->  CoMXYZ1" : Selector  NumberOfDimensions=2  InputPortWidth=7  IndexOptions=Index vector (dialog),Index vector (dialog)  Indices=[1 2 3],[1 2 3]  OutputSizes=1,1
  "CoM6D ->  CoMXYZ2" : Selector  NumberOfDimensions=2  InputPortWidth=7  IndexOptions=Index vector (dialog),Index vector (dialog)  Indices=[1 2 3],[4]  OutputSizes=1,1
  Hom : Scope
      settings: TimeRange=auto  LimitDataPoints=on  MaxDataPoints=5000  SaveToWorkspace=off  SaveName=ScopeData  YMin=-10  YMax=10  SampleTime=-1  DataFormat=Array
  R : Scope
      settings: TimeRange=auto  LimitDataPoints=on  MaxDataPoints=5000  SaveToWorkspace=off  SaveName=ScopeData  YMin=-10  YMax=10  SampleTime=-1  DataFormat=Array
  p : Scope
      settings: TimeRange=auto  LimitDataPoints=on  MaxDataPoints=5000  SaveToWorkspace=off  SaveName=ScopeData  YMin=-10  YMax=10  SampleTime=-1  DataFormat=Array
  wires:
  "CoM6D ->  CoMXYZ1"/1 -> R/1
  "CoM6D ->  CoMXYZ2"/1 -> p/1
  H/1 -> "CoM6D ->  CoMXYZ2"/1, Hom/1, "CoM6D ->  CoMXYZ1"/1

== system torqueBalancingR2015a/State Machine/State Machine Walking/visualise inertial/Visualize hom transf4 ==
  H : Inport
  "CoM6D ->  CoMXYZ1" : Selector  NumberOfDimensions=2  InputPortWidth=7  IndexOptions=Index vector (dialog),Index vector (dialog)  Indices=[1 2 3],[1 2 3]  OutputSizes=1,1
  "CoM6D ->  CoMXYZ2" : Selector  NumberOfDimensions=2  InputPortWidth=7  IndexOptions=Index vector (dialog),Index vector (dialog)  Indices=[1 2 3],[4]  OutputSizes=1,1
  Hom : Scope
      settings: TimeRange=auto  LimitDataPoints=on  MaxDataPoints=5000  SaveToWorkspace=off  SaveName=ScopeData  YMin=-10  YMax=10  SampleTime=-1  DataFormat=Array
  R : Scope
      settings: TimeRange=auto  LimitDataPoints=on  MaxDataPoints=5000  SaveToWorkspace=off  SaveName=ScopeData  YMin=-10  YMax=10  SampleTime=-1  DataFormat=Array
  p : Scope
      settings: TimeRange=auto  LimitDataPoints=on  MaxDataPoints=5000  SaveToWorkspace=off  SaveName=ScopeData  YMin=-10  YMax=10  SampleTime=-1  DataFormat=Array
  wires:
  "CoM6D ->  CoMXYZ1"/1 -> R/1
  "CoM6D ->  CoMXYZ2"/1 -> p/1
  H/1 -> "CoM6D ->  CoMXYZ2"/1, Hom/1, "CoM6D ->  CoMXYZ1"/1

== system torqueBalancingR2015a/State Machine/State Machine Walking/visualise inertial/Visualize hom transf5 ==
  H : Inport
  "CoM6D ->  CoMXYZ1" : Selector  NumberOfDimensions=2  InputPortWidth=7  IndexOptions=Index vector (dialog),Index vector (dialog)  Indices=[1 2 3],[1 2 3]  OutputSizes=1,1
  "CoM6D ->  CoMXYZ2" : Selector  NumberOfDimensions=2  InputPortWidth=7  IndexOptions=Index vector (dialog),Index vector (dialog)  Indices=[1 2 3],[4]  OutputSizes=1,1
  Hom : Scope
      settings: TimeRange=auto  LimitDataPoints=on  MaxDataPoints=5000  SaveToWorkspace=off  SaveName=ScopeData  YMin=-10  YMax=10  SampleTime=-1  DataFormat=Array
  R : Scope
      settings: TimeRange=auto  LimitDataPoints=on  MaxDataPoints=5000  SaveToWorkspace=off  SaveName=ScopeData  YMin=-10  YMax=10  SampleTime=-1  DataFormat=Array
  p : Scope
      settings: TimeRange=auto  LimitDataPoints=on  MaxDataPoints=5000  SaveToWorkspace=off  SaveName=ScopeData  YMin=-10  YMax=10  SampleTime=-1  DataFormat=Array
  wires:
  "CoM6D ->  CoMXYZ1"/1 -> R/1
  "CoM6D ->  CoMXYZ2"/1 -> p/1
  H/1 -> "CoM6D ->  CoMXYZ2"/1, Hom/1, "CoM6D ->  CoMXYZ1"/1

== system torqueBalancingR2015a/State Machine/State Machine Walking/visualise inertial/Visualize hom transf7 ==
  H : Inport
  "CoM6D ->  CoMXYZ1" : Selector  NumberOfDimensions=2  InputPortWidth=7  IndexOptions=Index vector (dialog),Index vector (dialog)  Indices=[1 2 3],[1 2 3]  OutputSizes=1,1
  "CoM6D ->  CoMXYZ2" : Selector  NumberOfDimensions=2  InputPortWidth=7  IndexOptions=Index vector (dialog),Index vector (dialog)  Indices=[1 2 3],[4]  OutputSizes=1,1
  Hom : Scope
      settings: TimeRange=auto  LimitDataPoints=on  MaxDataPoints=5000  SaveToWorkspace=off  SaveName=ScopeData  YMin=-10  YMax=10  SampleTime=-1  DataFormat=Array
  R : Scope
      settings: TimeRange=auto  LimitDataPoints=on  MaxDataPoints=5000  SaveToWorkspace=off  SaveName=ScopeData  YMin=-10  YMax=10  SampleTime=-1  DataFormat=Array
  p : Scope
      settings: TimeRange=auto  LimitDataPoints=on  MaxDataPoints=5000  SaveToWorkspace=off  SaveName=ScopeData  YMin=-10  YMax=10  SampleTime=-1  DataFormat=Array
  wires:
  "CoM6D ->  CoMXYZ1"/1 -> R/1
  "CoM6D ->  CoMXYZ2"/1 -> p/1
  H/1 -> "CoM6D ->  CoMXYZ2"/1, Hom/1, "CoM6D ->  CoMXYZ1"/1

== system torqueBalancingR2015a/State Machine/State Machine Walking/visualise inertial/l_sole_H_root_link1 ==
  qj : Inport
  Constant5 : Constant  Value=eye(4)
  Constant6 : Constant  Value=eye(4)
  Inv\* : Product  Inputs=/*  Multiplication=Matrix(*)
  Visualize hom transf7 : Subsystem
  link_name : WBToolboxLibrary/wholeBodyModel/Kinematics/Forward Kinematics  frameName=link_name  robotName=WBT_robotName  localName=WBT_modelName  wbiFile=WBT_wbiFilename  wbiList=WBT_wbiList
  root_link : WBToolboxLibrary/wholeBodyModel/Kinematics/Forward Kinematics  frameName=FRAMES.BASE  robotName=WBT_robotName  localName=WBT_modelName  wbiFile=WBT_wbiFilename  wbiList=WBT_wbiList
  link_name_H_root_link : Outport
  wires:
  Constant5/1 -> link_name/1
  Inv\*/1 -> link_name_H_root_link/1  "link_name_H_root_link"
  link_name/1 -> Inv\*/1
  Constant6/1 -> root_link/1
  qj/1 -> root_link/2, link_name/2
  root_link/1 -> Visualize hom transf7/1(H), Inv\*/2

== system torqueBalancingR2015a/State Machine/State Machine Walking/visualise inertial/l_sole_H_root_link2 ==
  qj : Inport
  Constant5 : Constant  Value=eye(4)
  Constant6 : Constant  Value=eye(4)
  Inv\* : Product  Inputs=/*  Multiplication=Matrix(*)
  Visualize hom transf7 : Subsystem
  link_name : WBToolboxLibrary/wholeBodyModel/Kinematics/Forward Kinematics  frameName=link_name  robotName=WBT_robotName  localName=WBT_modelName  wbiFile=WBT_wbiFilename  wbiList=WBT_wbiList
  root_link : WBToolboxLibrary/wholeBodyModel/Kinematics/Forward Kinematics  frameName=FRAMES.BASE  robotName=WBT_robotName  localName=WBT_modelName  wbiFile=WBT_wbiFilename  wbiList=WBT_wbiList
  link_name_H_root_link : Outport
  wires:
  Constant5/1 -> link_name/1
  Inv\*/1 -> link_name_H_root_link/1  "link_name_H_root_link"
  link_name/1 -> Inv\*/1
  Constant6/1 -> root_link/1
  qj/1 -> root_link/2, link_name/2
  root_link/1 -> Visualize hom transf7/1(H), Inv\*/2

== system torqueBalancingR2015a/State Machine/State Machine Walking/visualise inertial/w_H_root_link1 ==
  qj : Inport
  inertial : Inport  Port=2
  "CoM6D ->  CoMXYZ1" : Selector  NumberOfDimensions=2  InputPortWidth=7  IndexOptions=Index vector (dialog),Index vector (dialog)  Indices=[1 2 3],[1 2 3]  OutputSizes=1,1
  Constant2 : Constant  Value=eye(4)
  Constant5 : Constant  Value=eye(4)
  Constant6 : Constant  Value=eye(4)
  Inv\* : Product  Inputs=/*  Multiplication=Matrix(*)
  Inv\*1 : Product  Inputs=/*  Multiplication=Matrix(*)
  Inv\*2 : Product  Inputs=/  Multiplication=Matrix(*)
  Product : Product  Multiplication=Matrix(*)
  Selector : Selector  InputPortWidth=12  IndexOptions=Index vector (dialog)  Indices=[4 5 6 ]  OutputSizes=1
  Subsystem : Subsystem
  Switch6 : Switch  Criteria=u2 > Threshold
  USE_IMU4EST_BASE : Constant  Value=CONFIG.USE_IMU4EST_BASE
  fromImuToHomogeousTransformFCN : MATLAB Function  TreatAsAtomicUnit=on
      settings: PermitHierarchicalResolution=ParametersOnly
  holder 1 : WBToolboxLibrary/Utilities/holder 
  holder 2 : WBToolboxLibrary/Utilities/holder 
  imu : WBToolboxLibrary/wholeBodyModel/Kinematics/Forward Kinematics  frameName='imu_frame'  robotName=WBT_robotName  localName=WBT_modelName  wbiFile=WBT_wbiFilename  wbiList=WBT_wbiList
  l_sole_acc : Scope
      settings: TimeRange=auto  LimitDataPoints=on  MaxDataPoints=5000  SaveToWorkspace=off  SaveName=ScopeData  YMin=-10  YMax=10  SampleTime=-1  DataFormat=Array
  link : WBToolboxLibrary/wholeBodyModel/Kinematics/Forward Kinematics  frameName=link_name  robotName=WBT_robotName  localName=WBT_modelName  wbiFile=WBT_wbiFilename  wbiList=WBT_wbiList
  root_link : WBToolboxLibrary/wholeBodyModel/Kinematics/Forward Kinematics  frameName='root_link'  robotName=WBT_robotName  localName=WBT_modelName  wbiFile=WBT_wbiFilename  wbiList=WBT_wbiList
  w_H_root : Outport
  wires:
  Constant5/1 -> imu/1
  Inv\*/1 -> holder 1/1, fromImuToHomogeousTransformFCN/1(imu_H_link), Inv\*2/1  "imu_H_link"
  imu/1 -> Inv\*/1
  Constant6/1 -> link/1
  Inv\*1/1 -> Switch6/3, fromImuToHomogeousTransformFCN/3(link_H_root)  "link_H_root"
  link/1 -> Inv\*1/1, Inv\*/2
  inertial/1 -> Selector/1, holder 2/1, fromImuToHomogeousTransformFCN/5(inertial)
  Switch6/1 -> w_H_root/1
  USE_IMU4EST_BASE/1 -> Switch6/2
  fromImuToHomogeousTransformFCN/1(w_H_root) -> Switch6/1
  Constant2/1 -> root_link/1
  qj/1 -> root_link/2, link/2, imu/2
  root_link/1 -> Inv\*1/2
  holder 1/1 -> fromImuToHomogeousTransformFCN/2(imu_H_link_0)
  holder 2/1 -> fromImuToHomogeousTransformFCN/4(inertial_0)
  Inv\*2/1 -> "CoM6D ->  CoMXYZ1"/1
  "CoM6D ->  CoMXYZ1"/1 -> Product/1  "l_sole_R_imu"
  Selector/1 -> Product/2  "imu_acce"
  Product/1 -> l_sole_acc/1
  Subsystem/1(Neck Position) -> fromImuToHomogeousTransformFCN/6(neck)

== system torqueBalancingR2015a/State Machine/State Machine Walking/visualise inertial/w_H_root_link2 ==
  qj : Inport
  inertial : Inport  Port=2
  "CoM6D ->  CoMXYZ1" : Selector  NumberOfDimensions=2  InputPortWidth=7  IndexOptions=Index vector (dialog),Index vector (dialog)  Indices=[1 2 3],[1 2 3]  OutputSizes=1,1
  Constant2 : Constant  Value=eye(4)
  Constant5 : Constant  Value=eye(4)
  Constant6 : Constant  Value=eye(4)
  Inv\* : Product  Inputs=/*  Multiplication=Matrix(*)
  Inv\*1 : Product  Inputs=/*  Multiplication=Matrix(*)
  Inv\*2 : Product  Inputs=/  Multiplication=Matrix(*)
  Product : Product  Multiplication=Matrix(*)
  Selector : Selector  InputPortWidth=12  IndexOptions=Index vector (dialog)  Indices=[4 5 6 ]  OutputSizes=1
  Subsystem : Subsystem
  Switch6 : Switch  Criteria=u2 > Threshold
  USE_IMU4EST_BASE : Constant  Value=CONFIG.USE_IMU4EST_BASE
  fromImuToHomogeousTransformFCN : MATLAB Function  TreatAsAtomicUnit=on
      settings: PermitHierarchicalResolution=ParametersOnly
  holder 1 : WBToolboxLibrary/Utilities/holder 
  holder 2 : WBToolboxLibrary/Utilities/holder 
  imu : WBToolboxLibrary/wholeBodyModel/Kinematics/Forward Kinematics  frameName='imu_frame'  robotName=WBT_robotName  localName=WBT_modelName  wbiFile=WBT_wbiFilename  wbiList=WBT_wbiList
  l_sole_acc : Scope
      settings: TimeRange=auto  LimitDataPoints=on  MaxDataPoints=5000  SaveToWorkspace=off  SaveName=ScopeData  YMin=-10  YMax=10  SampleTime=-1  DataFormat=Array
  link : WBToolboxLibrary/wholeBodyModel/Kinematics/Forward Kinematics  frameName=link_name  robotName=WBT_robotName  localName=WBT_modelName  wbiFile=WBT_wbiFilename  wbiList=WBT_wbiList
  root_link : WBToolboxLibrary/wholeBodyModel/Kinematics/Forward Kinematics  frameName='root_link'  robotName=WBT_robotName  localName=WBT_modelName  wbiFile=WBT_wbiFilename  wbiList=WBT_wbiList
  w_H_root : Outport
  wires:
  Constant5/1 -> imu/1
  Inv\*/1 -> holder 1/1, fromImuToHomogeousTransformFCN/1(imu_H_link), Inv\*2/1  "imu_H_link"
  imu/1 -> Inv\*/1
  Constant6/1 -> link/1
  Inv\*1/1 -> Switch6/3, fromImuToHomogeousTransformFCN/3(link_H_root)  "link_H_root"
  link/1 -> Inv\*1/1, Inv\*/2
  inertial/1 -> Selector/1, holder 2/1, fromImuToHomogeousTransformFCN/5(inertial)
  Switch6/1 -> w_H_root/1
  USE_IMU4EST_BASE/1 -> Switch6/2
  fromImuToHomogeousTransformFCN/1(w_H_root) -> Switch6/1
  Constant2/1 -> root_link/1
  qj/1 -> root_link/2, link/2, imu/2
  root_link/1 -> Inv\*1/2
  holder 1/1 -> fromImuToHomogeousTransformFCN/2(imu_H_link_0)
  holder 2/1 -> fromImuToHomogeousTransformFCN/4(inertial_0)
  Inv\*2/1 -> "CoM6D ->  CoMXYZ1"/1
  "CoM6D ->  CoMXYZ1"/1 -> Product/1  "l_sole_R_imu"
  Selector/1 -> Product/2  "imu_acce"
  Product/1 -> l_sole_acc/1
  Subsystem/1(Neck Position) -> fromImuToHomogeousTransformFCN/6(neck)

== system torqueBalancingR2015a/State Machine/State Machine Yoga/visualise inertial/Visualize hom transf1 ==
  H : Inport
  "CoM6D ->  CoMXYZ1" : Selector  NumberOfDimensions=2  InputPortWidth=7  IndexOptions=Index vector (dialog),Index vector (dialog)  Indices=[1 2 3],[1 2 3]  OutputSizes=1,1
  "CoM6D ->  CoMXYZ2" : Selector  NumberOfDimensions=2  InputPortWidth=7  IndexOptions=Index vector (dialog),Index vector (dialog)  Indices=[1 2 3],[4]  OutputSizes=1,1
  Hom : Scope
      settings: TimeRange=auto  LimitDataPoints=on  MaxDataPoints=5000  SaveToWorkspace=off  SaveName=ScopeData  YMin=-10  YMax=10  SampleTime=-1  DataFormat=Array
  R : Scope
      settings: TimeRange=auto  LimitDataPoints=on  MaxDataPoints=5000  SaveToWorkspace=off  SaveName=ScopeData  YMin=-10  YMax=10  SampleTime=-1  DataFormat=Array
  p : Scope
      settings: TimeRange=auto  LimitDataPoints=on  MaxDataPoints=5000  SaveToWorkspace=off  SaveName=ScopeData  YMin=-10  YMax=10  SampleTime=-1  DataFormat=Array
  wires:
  "CoM6D ->  CoMXYZ1"/1 -> R/1
  "CoM6D ->  CoMXYZ2"/1 -> p/1
  H/1 -> "CoM6D ->  CoMXYZ2"/1, Hom/1, "CoM6D ->  CoMXYZ1"/1

== system torqueBalancingR2015a/State Machine/State Machine Yoga/visualise inertial/Visualize hom transf2 ==
  H : Inport
  "CoM6D ->  CoMXYZ1" : Selector  NumberOfDimensions=2  InputPortWidth=7  IndexOptions=Index vector (dialog),Index vector (dialog)  Indices=[1 2 3],[1 2 3]  OutputSizes=1,1
  "CoM6D ->  CoMXYZ2" : Selector  NumberOfDimensions=2  InputPortWidth=7  IndexOptions=Index vector (dialog),Index vector (dialog)  Indices=[1 2 3],[4]  OutputSizes=1,1
  Hom : Scope
      settings: TimeRange=auto  LimitDataPoints=on  MaxDataPoints=5000  SaveToWorkspace=off  SaveName=ScopeData  YMin=-10  YMax=10  SampleTime=-1  DataFormat=Array
  R : Scope
      settings: TimeRange=auto  LimitDataPoints=on  MaxDataPoints=5000  SaveToWorkspace=off  SaveName=ScopeData  YMin=-10  YMax=10  SampleTime=-1  DataFormat=Array
  p : Scope
      settings: TimeRange=auto  LimitDataPoints=on  MaxDataPoints=5000  SaveToWorkspace=off  SaveName=ScopeData  YMin=-10  YMax=10  SampleTime=-1  DataFormat=Array
  wires:
  "CoM6D ->  CoMXYZ1"/1 -> R/1
  "CoM6D ->  CoMXYZ2"/1 -> p/1
  H/1 -> "CoM6D ->  CoMXYZ2"/1, Hom/1, "CoM6D ->  CoMXYZ1"/1

== system torqueBalancingR2015a/State Machine/State Machine Yoga/visualise inertial/Visualize hom transf3 ==
  H : Inport
  "CoM6D ->  CoMXYZ1" : Selector  NumberOfDimensions=2  InputPortWidth=7  IndexOptions=Index vector (dialog),Index vector (dialog)  Indices=[1 2 3],[1 2 3]  OutputSizes=1,1
  "CoM6D ->  CoMXYZ2" : Selector  NumberOfDimensions=2  InputPortWidth=7  IndexOptions=Index vector (dialog),Index vector (dialog)  Indices=[1 2 3],[4]  OutputSizes=1,1
  Hom : Scope
      settings: TimeRange=auto  LimitDataPoints=on  MaxDataPoints=5000  SaveToWorkspace=off  SaveName=ScopeData  YMin=-10  YMax=10  SampleTime=-1  DataFormat=Array
  R : Scope
      settings: TimeRange=auto  LimitDataPoints=on  MaxDataPoints=5000  SaveToWorkspace=off  SaveName=ScopeData  YMin=-10  YMax=10  SampleTime=-1  DataFormat=Array
  p : Scope
      settings: TimeRange=auto  LimitDataPoints=on  MaxDataPoints=5000  SaveToWorkspace=off  SaveName=ScopeData  YMin=-10  YMax=10  SampleTime=-1  DataFormat=Array
  wires:
  "CoM6D ->  CoMXYZ1"/1 -> R/1
  "CoM6D ->  CoMXYZ2"/1 -> p/1
  H/1 -> "CoM6D ->  CoMXYZ2"/1, Hom/1, "CoM6D ->  CoMXYZ1"/1
